simulink model "LAB3_Euler_eq_with_rotor"  (R2022b)
settings: Solver=ode5  StartTime=0.0  StopTime=100  FixedStep=0.1  RelTol=1e-3
values from neighbouring files (symbols this model uses):
  Ir = [0 0 0; 0 0 0; 0 0 0.005]    [LAB_03.m]
  Is = diag([0.07 , 0.055 , 0.025])    [LAB_03.m]
  Mr = [ 0 ; 0 ; 0]    [LAB_03.m]
  wr_0 = [ 0 , 0 , 2*pi]    [LAB_03.m]
  ws_0 = [1e-6 , 1e-6 , 0.02]    [LAB_03.m]
libraries: matrix_library x1
settings Model: Creator=ludov  LastModifiedBy=ludov

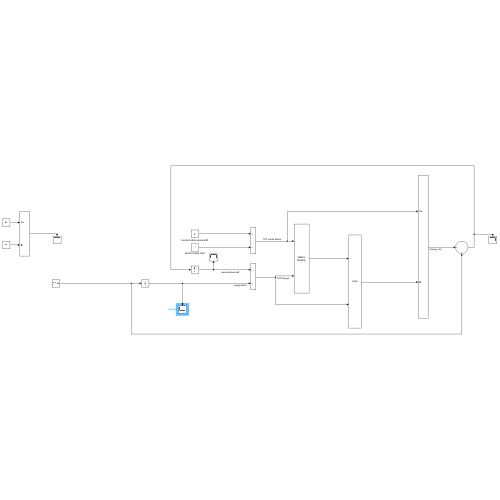
[thumbnail: Simulink's stored preview of the top-level diagram]
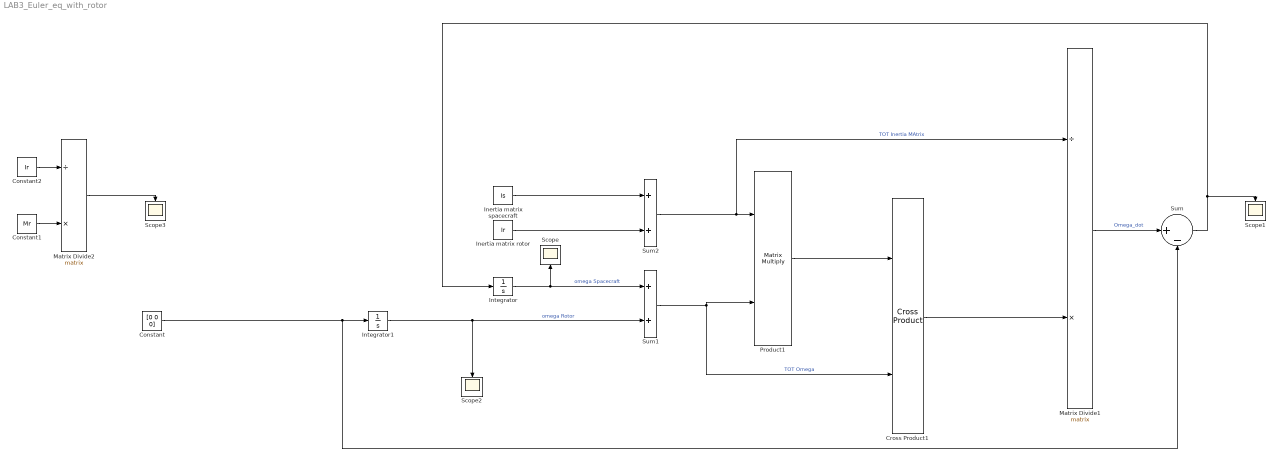
== system LAB3_Euler_eq_with_rotor ==
  Constant : Constant  Value=[0 0 0]
  Constant1 : Constant  Value=Mr
  Constant2 : Constant  Value=Ir
  Cross Product1 : matrix_library/Cross Product
  Inertia matrix rotor : Constant  Value=Ir
  Inertia matrix spacecraft : Constant  Value=Is
  Integrator : Integrator  InitialCondition=ws_0
  Integrator1 : Integrator  InitialCondition=wr_0
  Matrix Divide1 : Product  Inputs=/*  Multiplication=Matrix(*)
  Matrix Divide2 : Product  Inputs=/*  Multiplication=Matrix(*)
  Product1 : Product  Multiplication=Matrix(*)
  Scope{,1..3} (4 alike) : Scope
  Sum : Sum  Inputs=|+-
  Sum1 : Sum
  Sum2 : Sum
  wires:
  Inertia matrix spacecraft/1 -> Sum2/1
  Inertia matrix rotor/1 -> Sum2/2
  Sum2/1 -> Matrix Divide1/1, Product1/1  "TOT Inertia MAtrix"
  Sum1/1 -> Product1/2, Cross Product1/2  "TOT Omega"
  Integrator1/1 -> Scope2/1, Sum1/2  "omega Rotor"
  Integrator/1 -> Scope/1, Sum1/1  "omega Spacecraft"
  Product1/1 -> Cross Product1/1
  Cross Product1/1 -> Matrix Divide1/2
  Constant2/1 -> Matrix Divide2/1
  Constant1/1 -> Matrix Divide2/2
  Sum/1 -> Scope1/1, Integrator/1
  Constant/1 -> Sum/2, Integrator1/1
  Matrix Divide1/1 -> Sum/1  "Omega_dot"
  Matrix Divide2/1 -> Scope3/1
